simulink model "three_body_PID"  (R2023b)
settings: Solver=ode4  StartTime=0.0  StopTime=20  FixedStep=0.001  RelTol=1e-3
values from neighbouring files (symbols this model uses):
  dot_X0 = trajectory(1, 4:5)    [init.m]
  trajectory = readmatrix("trajectory.csv")    [init.m]
  X0 = trajectory(1, 1:2)    [init.m]
undefined symbols (not defined in the file or in its folder): mu
libraries: slpidlib x1
settings Model: Creator=Ali  LastModifiedBy=Ali

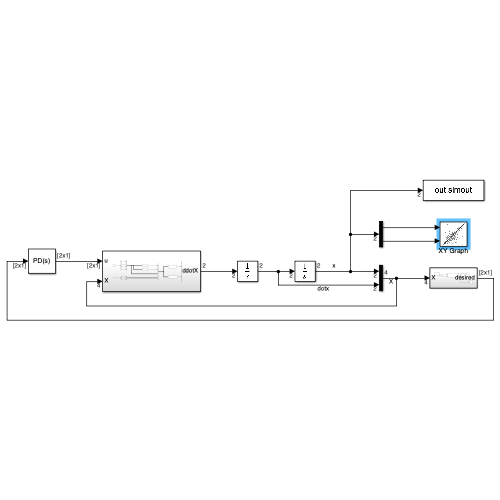
[thumbnail: Simulink's stored preview of the top-level diagram]
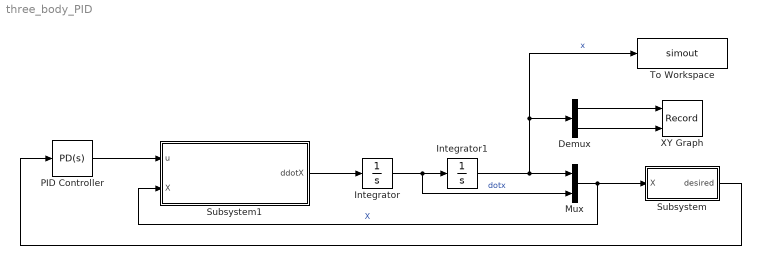
== system three_body_PID ==
  Demux : Demux  Outputs=2
  Integrator : Integrator  InitialCondition=dot_X0
  Integrator1 : Integrator  InitialCondition=X0
  Mux : Mux  Inputs=2
  PID Controller : slpidlib/PID Controller  Controller=PD  Form=Parallel  TimeDomain=Continuous-time  UseExternalTs=off  SampleTime=-1  IntegratorMethod=Forward Euler  FilterMethod=Forward Euler  ControllerParametersSource=internal  P=10  I=0  UseKiTs=off  D=0  N=100  UseFilter=on  TunerSelectOption=Transfer Function Based (PID Tuner App)  InitialConditionSource=internal  InitialConditionForIntegrator=0  InitialConditionForFilter=0  DifferentiatorICPrevScaledInput=0  ExternalReset=none  TrackingMode=off  Kt=1  LimitOutput=off  SatLimitsSource=internal  UpperSaturationLimit=inf  LowerSaturationLimit=-inf  LinearizeAsGain=on  AntiWindupMode=none  Kb=1  LimitIntegrator=off  UpperIntegratorSaturationLimit=inf  LowerIntegratorSaturationLimit=-inf  POutMin=[]  POutMax=[]  IOutMin=[]  IOutMax=[]  DOutMin=[]  DOutMax=[]  NOutMin=[]  NOutMax=[]  SumOutMin=[]  SumOutMax=[]  SaturationOutMin=[]  SaturationOutMax=[]  PParamMin=[]  PParamMax=[]  IParamMin=[]  IParamMax=[]  DParamMin=[]  DParamMax=[]  NParamMin=[]  NParamMax=[]  KbParamMin=[]  KbParamMax=[]  KtParamMin=[]  KtParamMax=[]  KbOutMin=[]  KbOutMax=[]  KtOutMin=[]  KtOutMax=[]  IntegratorOutMin=[]  IntegratorOutMax=[]  FilterOutMin=[]  FilterOutMax=[]  SumI1OutMin=[]  SumI1OutMax=[]  SumI2OutMin=[]  SumI2OutMax=[]  SumI3OutMin=[]  SumI3OutMax=[]  SumI4OutMin=[]  SumI4OutMax=[]  SumDOutMin=[]  SumDOutMax=[]  DifferentiatorOutMin=[]  DifferentiatorOutMax=[]  FilterDiffOutCoefMin=[]  FilterDiffOutCoefMax=[]  ReciprocalOutMin=[]  ReciprocalOutMax=[]  SumDenOutMin=[]  SumDenOutMax=[]  SumNumOutMin=[]  SumNumOutMax=[]  DivideOutMin=[]  DivideOutMax=[]  UdiffTsProdOutMin=[]  UdiffTsProdOutMax=[]  NTsProdOutMin=[]  NTsProdOutMax=[]  UintegralTsProdOutMin=[]  UintegralTsProdOutMax=[]  UngainTsProdOutMin=[]  UngainTsProdOutMax=[]  ClampingZeroOutDataTypeStr=Inherit: Inherit via back propagation  ClampingZeroOutMin=[]  ClampingZeroOutMax=[]  FilterDenConstantOutDataTypeStr=Inherit: Inherit via back propagation  FilterDenConstantOutMin=[]  FilterDenConstantOutMax=[]  PCopyOutDataTypeStr=Inherit: Inherit via back propagation  PCopyOutMin=[]  PCopyOutMax=[]  NCopyOutDataTypeStr=Inherit: Inherit via back propagation  NCopyOutMin=[]  NCopyOutMax=[]  IntegratorContinuousStateAttributes=''  IntegratorStateMustResolveToSignalObject=off  IntegratorRTWStateStorageClass=Auto  FilterContinuousStateAttributes=''  FilterStateMustResolveToSignalObject=off  FilterRTWStateStorageClass=Auto  ParallelPVariant=InternalParameters  IdealPVariant=Disabled  IVariant=Disabled  DVariant=InternalParameters  IntegratorVariant=Disabled  SatVariant=Disabled  AWVariant=Disabled  PCopyVariant=Disabled  TRVariant=Disabled  FdbkBlocksVariant=Forward  IdealPFdbkVariant=Disabled  SatFdbkVariant=Disabled  DerivativeFilterVariant=ContFilter  NVariant=InternalParameters  NCopyVariant=Disabled  FilterICVariant=InternalICsFilter  IntegratorICVariant=Disabled  ExternalResetVariant=Disabled  TRSumVariant=Passthrough  SumFdbkVariant=Disabled  SumVariant=Sum_PD  TsampFilterVariant=InternalTs  TsampNgainVariant=Passthrough  TsampIntegralVariant=Disabled_SignalSpec  ExternalSaturationOutDataTypeStr=Inherit: Same as second input
  Subsystem : Subsystem
  Subsystem1 : Subsystem
  To Workspace : ToWorkspace  VariableName=simout  SampleTime=-1
      settings: Save2DSignal=2-D array (concatenate along first dimension)
  XY Graph : Record  FileSettingsInternal="{\"entries\":[{\"content\":{\"excelSettings\":{\"content\":{},\"type\":\"Streamout.ExcelSettings\"}},\"type\":\"Streamout.FileSettingStorage\",\"uuid\":\"\"}],\"packageUris\":[\"http:\\/\\/schema.mathworks.com\\/mf0\\/streamout_blocks\\/R2020a\"],\"version\":\"1.0\"}"  Layout=[1 1]  SignalsInternal="{\"entries\":[{\"content\":{\"signals\":[{\"content\":{\"blockPath\":[],\"dimensions\":[1],\"domain\":\"\",\"lineColor\":\"#a2142f\",\"plots\":[1],\"port\":1,\"sid\":[\"\"],\"signalID\":10867,\"signalName\":\"Demux:1\"},\"type\":\"RecordBlkView.Signal\",\"uuid\":\"\"},{\"content\":{\"blockPath\":[],\"dimensions\":[1],\"domain\":\"\",\"lineColor\":\"#139fff\",\"plots\":[1],\"port\":2,\"sid\":[\"\"],\"signalID\":10871,\"signalName\":\"Demux:2\"},\"type\":\"RecordBlkView.Signal\",\"uuid\":\"\"}]},\"type\":\"RecordBlkView.InputSignals\",\"uuid\":\"\"}],\"packageUris\":[\"http:\\/\\/schema.mathworks.com\\/mf0\\/streamout_blocks\\/R2020a\"],\"version\":\"1.0\"}"  VisualizationBindings="{\"xyplotplugin\":{\"info\":[{\"series\":[{\"bindingParametersList\":[{\"parameter\":\"X-Axis\",\"signalID\":10867,\"signalName\":\"Demux:1\"},{\"parameter\":\"Y-Axis\",\"signalID\":10871,\"signalName\":\"Demux:2\"}],\"seriesID\":19812}],\"subplotID\":1}]}}"  CompatibilityTag=XY
  wires:
  Integrator1/1 -> To Workspace/1, Demux/1, Mux/1  "x"
  Demux/1 -> XY Graph/1
  Demux/2 -> XY Graph/2
  Mux/1 -> Subsystem1/2(X), Subsystem/1(X)  "X"
  Integrator/1 -> Mux/2, Integrator1/1  "dotx"
  Subsystem/1(desired) -> PID Controller/1
  PID Controller/1 -> Subsystem1/1(u)
  Subsystem1/1(ddotX) -> Integrator/1

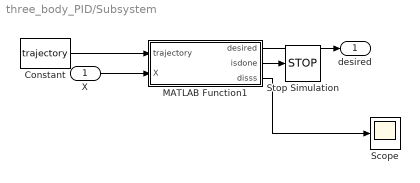
== system three_body_PID/Subsystem ==
  X : Inport
  Constant : Constant  Value=trajectory
  MATLAB Function1 : MATLAB Function  TreatAsAtomicUnit=on
  Scope : Scope
  Stop Simulation : Stop
  desired : Outport
  wires:
  MATLAB Function1/1(desired) -> desired/1
  Constant/1 -> MATLAB Function1/1(trajectory)
  X/1 -> MATLAB Function1/2(X)
  MATLAB Function1/3(disss) -> Scope/1
  MATLAB Function1/2(isdone) -> Stop Simulation/1

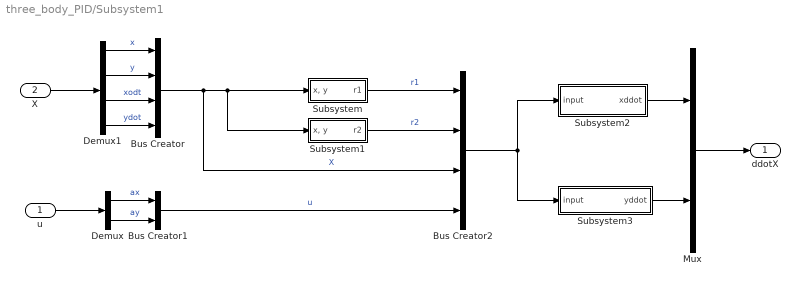
== system three_body_PID/Subsystem1 ==
  u : Inport
  X : Inport  Port=2
  Bus Creator : BusCreator  Inputs=4
  Bus Creator1 : BusCreator  Inputs=2
  Bus Creator2 : BusCreator  Inputs=4
  Demux : Demux  Outputs=2
  Demux1 : Demux
  Mux : Mux  Inputs=2
  Subsystem : Subsystem
  Subsystem1 : Subsystem
  Subsystem2 : Subsystem
  Subsystem3 : Subsystem
  ddotX : Outport
  wires:
  X/1 -> Demux1/1
  u/1 -> Demux/1
  Demux1/1 -> Bus Creator/1  "x"
  Demux1/2 -> Bus Creator/2  "y"
  Demux1/3 -> Bus Creator/3  "xodt"
  Demux1/4 -> Bus Creator/4  "ydot"
  Bus Creator/1 -> Bus Creator2/3, Subsystem1/1("x, y"), Subsystem/1("x, y")  "X"
  Subsystem/1(r1) -> Bus Creator2/1  "r1"
  Subsystem1/1(r2) -> Bus Creator2/2  "r2"
  Demux/1 -> Bus Creator1/1  "ax"
  Demux/2 -> Bus Creator1/2  "ay"
  Bus Creator1/1 -> Bus Creator2/4  "u"
  Bus Creator2/1 -> Subsystem3/1(input), Subsystem2/1(input)
  Subsystem2/1(xddot) -> Mux/1
  Subsystem3/1(yddot) -> Mux/2
  Mux/1 -> ddotX/1

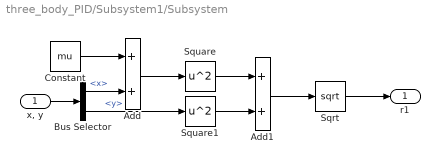
== system three_body_PID/Subsystem1/Subsystem ==
  "x, y" : Inport
  Add : Sum
  Add1 : Sum
  Bus Selector : BusSelector  OutputSignals=x,y
  Constant : Constant  Value=mu
  Sqrt : Sqrt
  Square : Math  Operator=square
  Square1 : Math  Operator=square
  r1 : Outport
  wires:
  Constant/1 -> Add/1
  Sqrt/1 -> r1/1
  Add/1 -> Square/1
  "x, y"/1 -> Bus Selector/1
  Add1/1 -> Sqrt/1
  Square1/1 -> Add1/2
  Square/1 -> Add1/1
  Bus Selector/1 -> Add/2  "<x>"
  Bus Selector/2 -> Square1/1  "<y>"

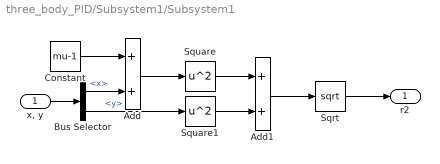
== system three_body_PID/Subsystem1/Subsystem1 ==
  "x, y" : Inport
  Add : Sum
  Add1 : Sum
  Bus Selector : BusSelector  OutputSignals=x,y
  Constant : Constant  Value=mu-1
  Sqrt : Sqrt
  Square : Math  Operator=square
  Square1 : Math  Operator=square
  r2 : Outport
  wires:
  Constant/1 -> Add/1
  Sqrt/1 -> r2/1
  Add/1 -> Square/1
  "x, y"/1 -> Bus Selector/1
  Add1/1 -> Sqrt/1
  Square1/1 -> Add1/2
  Square/1 -> Add1/1
  Bus Selector/1 -> Add/2  "<x>"
  Bus Selector/2 -> Square1/1  "<y>"

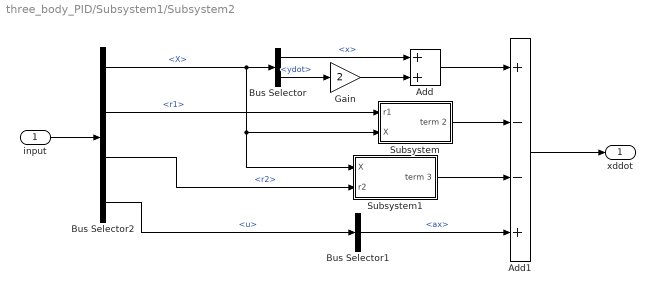
== system three_body_PID/Subsystem1/Subsystem2 ==
  input : Inport
  Add : Sum
  Add1 : Sum  Inputs=+--+
  Bus Selector : BusSelector  OutputSignals=x,ydot
  Bus Selector1 : BusSelector  OutputSignals=ax
  Bus Selector2 : BusSelector  OutputSignals=X,r1,r2,u
  Gain : Gain  Gain=2
  Subsystem : Subsystem
  Subsystem1 : Subsystem
  xddot : Outport
  wires:
  Bus Selector2/1 -> Bus Selector/1, Subsystem1/1(X), Subsystem/2(X)  "<X>"
  Bus Selector/1 -> Add/1  "<x>"
  Bus Selector/2 -> Gain/1  "<ydot>"
  Gain/1 -> Add/2
  Bus Selector2/2 -> Subsystem/1(r1)  "<r1>"
  Bus Selector2/3 -> Subsystem1/2(r2)  "<r2>"
  Bus Selector2/4 -> Bus Selector1/1  "<u>"
  Add/1 -> Add1/1
  Subsystem1/1(term 3) -> Add1/3
  Subsystem/1(term 2) -> Add1/2
  Bus Selector1/1 -> Add1/4  "<ax>"
  Add1/1 -> xddot/1
  input/1 -> Bus Selector2/1

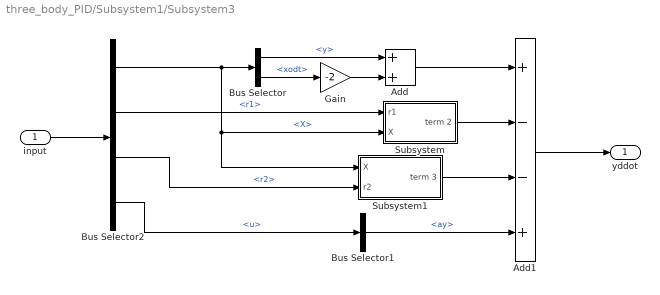
== system three_body_PID/Subsystem1/Subsystem3 ==
  input : Inport
  Add : Sum
  Add1 : Sum  Inputs=+--+
  Bus Selector : BusSelector  OutputSignals=y,xodt
  Bus Selector1 : BusSelector  OutputSignals=ay
  Bus Selector2 : BusSelector  OutputSignals=X,r1,r2,u
  Gain : Gain  Gain=-2
  Subsystem : Subsystem
  Subsystem1 : Subsystem
  yddot : Outport
  wires:
  Bus Selector2/1 -> Subsystem1/1(X), Subsystem/2(X), Bus Selector/1  "<X>"
  Bus Selector/1 -> Add/1  "<y>"
  Bus Selector/2 -> Gain/1  "<xodt>"
  Gain/1 -> Add/2
  Bus Selector2/2 -> Subsystem/1(r1)  "<r1>"
  Bus Selector2/3 -> Subsystem1/2(r2)  "<r2>"
  Bus Selector2/4 -> Bus Selector1/1  "<u>"
  Add/1 -> Add1/1
  Subsystem1/1(term 3) -> Add1/3
  Subsystem/1(term 2) -> Add1/2
  Bus Selector1/1 -> Add1/4  "<ay>"
  Add1/1 -> yddot/1
  input/1 -> Bus Selector2/1

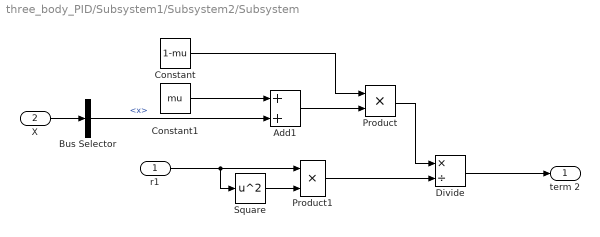
== system three_body_PID/Subsystem1/Subsystem2/Subsystem ==
  r1 : Inport
  X : Inport  Port=2
  Add1 : Sum
  Bus Selector : BusSelector  OutputSignals=x
  Constant : Constant  Value=1-mu
  Constant1 : Constant  Value=mu
  Divide : Product  Inputs=*/
  Product : Product
  Product1 : Product
  Square : Math  Operator=square
  term 2 : Outport
  wires:
  Square/1 -> Product1/2
  Product/1 -> Divide/1
  Add1/1 -> Product/2
  Constant/1 -> Product/1
  Constant1/1 -> Add1/1
  Divide/1 -> term 2/1
  r1/1 -> Product1/1, Square/1
  Product1/1 -> Divide/2
  X/1 -> Bus Selector/1
  Bus Selector/1 -> Add1/2  "<x>"

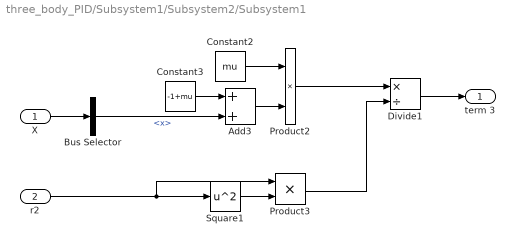
== system three_body_PID/Subsystem1/Subsystem2/Subsystem1 ==
  X : Inport
  r2 : Inport  Port=2
  Add3 : Sum
  Bus Selector : BusSelector  OutputSignals=x
  Constant2 : Constant  Value=mu
  Constant3 : Constant  Value=-1+mu
  Divide1 : Product  Inputs=*/
  Product2 : Product
  Product3 : Product
  Square1 : Math  Operator=square
  term 3 : Outport
  wires:
  Product3/1 -> Divide1/2
  Constant2/1 -> Product2/1
  Divide1/1 -> term 3/1
  Square1/1 -> Product3/2
  Add3/1 -> Product2/2
  Product2/1 -> Divide1/1
  Constant3/1 -> Add3/1
  r2/1 -> Square1/1, Product3/1
  X/1 -> Bus Selector/1
  Bus Selector/1 -> Add3/2  "<x>"

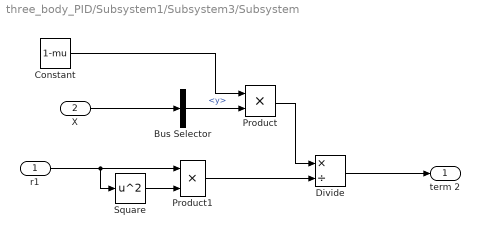
== system three_body_PID/Subsystem1/Subsystem3/Subsystem ==
  r1 : Inport
  X : Inport  Port=2
  Bus Selector : BusSelector  OutputSignals=y
  Constant : Constant  Value=1-mu
  Divide : Product  Inputs=*/
  Product : Product
  Product1 : Product
  Square : Math  Operator=square
  term 2 : Outport
  wires:
  Square/1 -> Product1/2
  Product/1 -> Divide/1
  Constant/1 -> Product/1
  Divide/1 -> term 2/1
  r1/1 -> Product1/1, Square/1
  Product1/1 -> Divide/2
  X/1 -> Bus Selector/1
  Bus Selector/1 -> Product/2  "<y>"

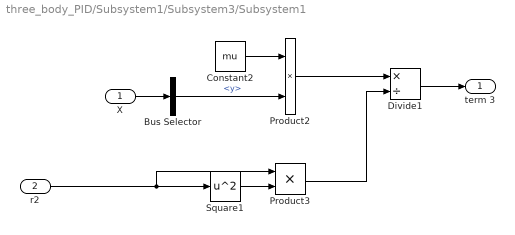
== system three_body_PID/Subsystem1/Subsystem3/Subsystem1 ==
  X : Inport
  r2 : Inport  Port=2
  Bus Selector : BusSelector  OutputSignals=y
  Constant2 : Constant  Value=mu
  Divide1 : Product  Inputs=*/
  Product2 : Product
  Product3 : Product
  Square1 : Math  Operator=square
  term 3 : Outport
  wires:
  Product3/1 -> Divide1/2
  Constant2/1 -> Product2/1
  Divide1/1 -> term 3/1
  Square1/1 -> Product3/2
  Product2/1 -> Divide1/1
  r2/1 -> Square1/1, Product3/1
  X/1 -> Bus Selector/1
  Bus Selector/1 -> Product2/2  "<y>"

== matlab function three_body_PID/Subsystem/MATLAB Function1 ==
  settings: updateMethod=DISCRETE
  data: trajectory input; desired output size=[2, 1]; X input; isdone output; disss output
function [desired, isdone, disss] = fcn(trajectory, X)

persistent point_index
if isempty(point_index)
    point_index = 0;
end

trajectory = trajectory(:, 1:2)';
xy = X(1:2);
distance = ((trajectory - xy).^2);
dist = sum(distance);
dist = dist';
index = find(dist==min(dist));
index = index(1);
if index <= point_index && index < length(trajectory)
    index = point_index + 1;
end
point_index = index;
if index > length(trajectory)
    index = length(trajectory);
end
answer = trajectory(:, index);
t = reshape(xy, [2, 1]);
desired = reshape(answer, [2, 1]) - t;
desired = desired * 100;

isdone = false;
final_point = trajectory(:, end);
disss = sqrt(sum((xy - final_point).^2));
if disss <= 0.005
    isdone = true;
end
